simulink model "ClosedObvTest"  (R2019b)
settings: Solver=VariableStepAuto  StartTime=0.0  StopTime=10.0  RelTol=1e-3
settings Model: Creator=jigarjhankharia  LastModifiedBy=aarij
settings DataIOCC: ReturnWorkspaceOutputs=off
settings DebuggingCC: ArithmeticOperatorsInVariantConditions=warning
settings SFSimCC: CustomCodeUndefinedFunction=UseInterfaceOnly

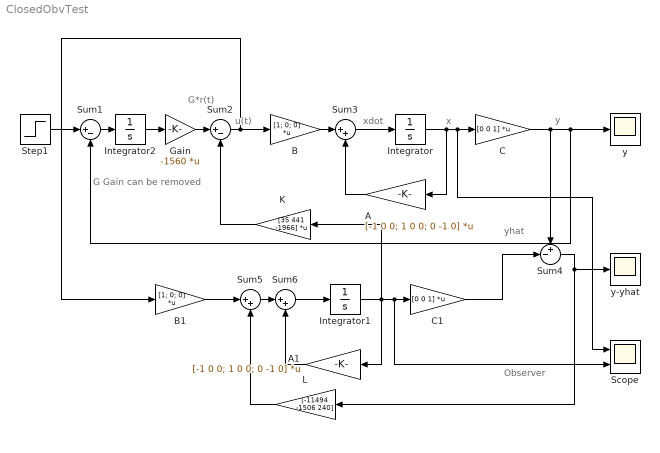
== system ClosedObvTest ==
  note: u(t)
  note: G*r(t)
  note: y
  note: xdot
  note: yhat
  note: x
  note: Observer
  note: G Gain can be removed
  A : Gain  Gain=[-1 0 0; 1 0 0; 0 -1 0]  Multiplication=Matrix(K*u) (u vector)
  A1 : Gain  Gain=[-1 0 0; 1 0 0; 0 -1 0]  Multiplication=Matrix(K*u) (u vector)
  B : Gain  Gain=[1; 0; 0]  Multiplication=Matrix(K*u) (u vector)
  B1 : Gain  Gain=[1; 0; 0]  Multiplication=Matrix(K*u) (u vector)
  C : Gain  Gain=[0 0 1]  Multiplication=Matrix(K*u) (u vector)
  C1 : Gain  Gain=[0 0 1]  Multiplication=Matrix(K*u) (u vector)
  Gain : Gain  Gain=-1560  Multiplication=Matrix(K*u)
  Integrator : Integrator  InitialCondition=[0 0 0 ]
  Integrator1 : Integrator  InitialCondition=[0 0 0]
  Integrator2 : Integrator
  K : Gain  Gain=[35 441 -1966]  Multiplication=Matrix(K*u) (u vector)
  L : Gain  Gain=[-11494 -1506 240]
  Scope : Scope  NumInputPorts=2
  Step1 : Step  Time=0  SampleTime=0
  Sum1 : Sum  Inputs=|+-
  Sum2 : Sum  Inputs=|+-
  Sum3 : Sum  Inputs=|++
  Sum4 : Sum  Inputs=+-|
  Sum5 : Sum  Inputs=|++
  Sum6 : Sum  Inputs=|++
  y : Scope
  y-yhat : Scope
  wires:
  B/1 -> Sum3/1
  Sum3/1 -> Integrator/1
  C/1 -> Sum4/1, Sum1/2, y/1
  Integrator/1 -> Scope/1, C/1, A/1
  C1/1 -> Sum4/2
  Sum2/1 -> B1/1, B/1
  B1/1 -> Sum5/1
  Sum5/1 -> Sum6/1
  A1/1 -> Sum6/2
  Sum6/1 -> Integrator1/1
  Integrator1/1 -> K/1, Scope/2, C1/1, A1/1
  L/1 -> Sum5/2
  Sum4/1 -> y-yhat/1, L/1
  A/1 -> Sum3/2
  K/1 -> Sum2/2
  Integrator2/1 -> Gain/1
  Gain/1 -> Sum2/1
  Step1/1 -> Sum1/1
  Sum1/1 -> Integrator2/1
